simulink model "problem5"  (R2025b)
settings: Solver=VariableStepAuto  StartTime=0.0  StopTime=10.0  RelTol=1e-3
settings Model: Creator=Maria Islam  LastModifiedBy=Maria Islam

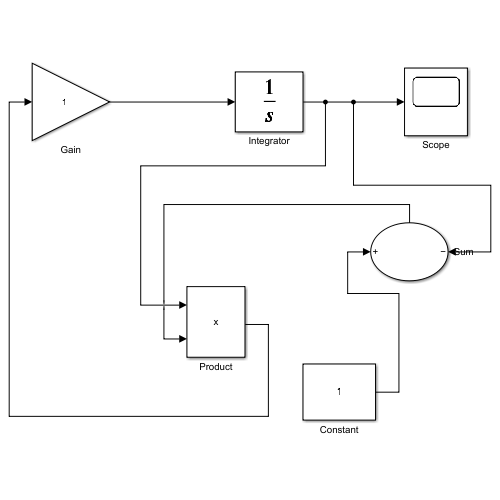
[thumbnail: Simulink's stored preview of the top-level diagram]
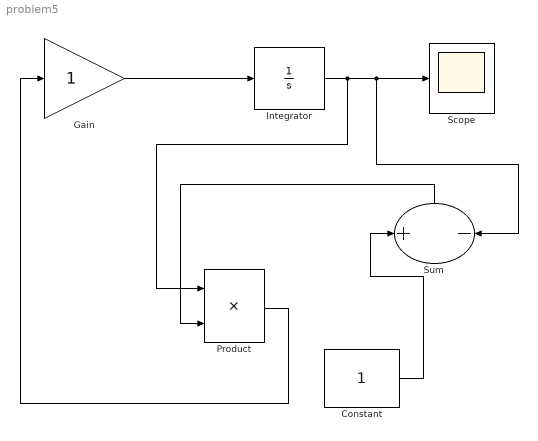
== system problem5 ==
  Constant : Constant
  Gain : Gain
  Integrator : Integrator  InitialCondition=0.1
  Product : Product
  Scope : Scope
      settings: ActiveDisplayYMinimum=-0.0475502415074221  ActiveDisplayYMaximum=1.0932640307529464
  Sum : Sum  Inputs=+-
  wires:
  Gain/1 -> Integrator/1
  Sum/1 -> Product/2
  Integrator/1 -> Product/1, Sum/2, Scope/1
  Constant/1 -> Sum/1
  Product/1 -> Gain/1
